simulink model "KalmanFilters"  (R2019b)
settings: Solver=FixedStepAuto  StartTime=0.0  StopTime=26.9950  FixedStep=0.005  RelTol=1e-3
InitFcn:
  | load('BusDefinitions.mat')
values from neighbouring files (symbols this model uses):
  M = [1 1 1 1 ... (first row only)    [parrot copy.m]
  q1 = 19.0085    [parrot copy.m]
  q2 = 5.761    [parrot copy.m]
  q3 = 15.4224    [parrot copy.m]
  q4 = 1.4190    (= 1.419)    [parrot copy.m]
  q5 = 6.1085    [parrot copy.m]
  r1 = .0731    (= 0.0731)    [parrot copy.m]
  r2 = 4.9726e+03    (= 4972.6)    [parrot copy.m]
  r3 = 7.7884e+03    (= 7788.4)    [parrot copy.m]
  r4 = .0160    (= 0.016)    [parrot copy.m]
  r5 = 3.0877    [parrot copy.m]
undefined symbols (not defined in the file or in its folder): codertarget, DiscIntNeverNeededParam, Discrete, Time
libraries: ctrlSharedLib x5
settings Model: ExtModeTrigDuration=80  Creator=The MathWorks, Inc.  LastModifiedBy=jockabethponce
settings DataIOCC: ReturnWorkspaceOutputs=off
settings OptimizationCC: PassReuseOutputArgsThreshold=0  MaxStackSize=64
settings DebuggingCC: ParameterTunabilityLossMsg=error  PregeneratedLibrarySubsystemCodeDiagnostic=none  ArithmeticOperatorsInVariantConditions=warning
settings HardwareCC: ProdBitPerPointer=32  ProdBitPerSizeT=32  ProdBitPerPtrDiffT=32  ProdLargestAtomicInteger=Long  ProdWordSize=32  ProdHWDeviceType=ARM Compatible->ARM 9
settings SFSimCC: SimUseLocalCustomCode=off  MATLABDynamicMemAlloc=off  CustomCodeUndefinedFunction=UseInterfaceOnly
settings RTWCC: SystemTargetFile=ert.tlc  HardwareBoard=PARROT Mambo  TLCOptions=-aInlineSetEventsForThisBaseRateFcn=TLC_FALSE -aSuppressMultiTaskScheduler=TLC_FALSE -aRateBasedStepFcn=1  TemplateMakefile=ert_default_tmf  GenerateReport=on  RTWUseLocalCustomCode=off  Toolchain=Sourcery G++ Lite GNU Toolchain for Drones  BuildConfiguration=Specify  LaunchReport=on
settings CodeAppCC: ForceParamTrailComments=on  OperatorAnnotations=on  StateflowObjectComments=on
settings ERTTargetCC: ERTCustomFileBanners=off  MatFileLogging=on  SupportContinuousTime=on  SupportNonInlinedSFcns=on  RemoveResetFunc=off  ModelStepFunctionPrototypeControlCompliant=off

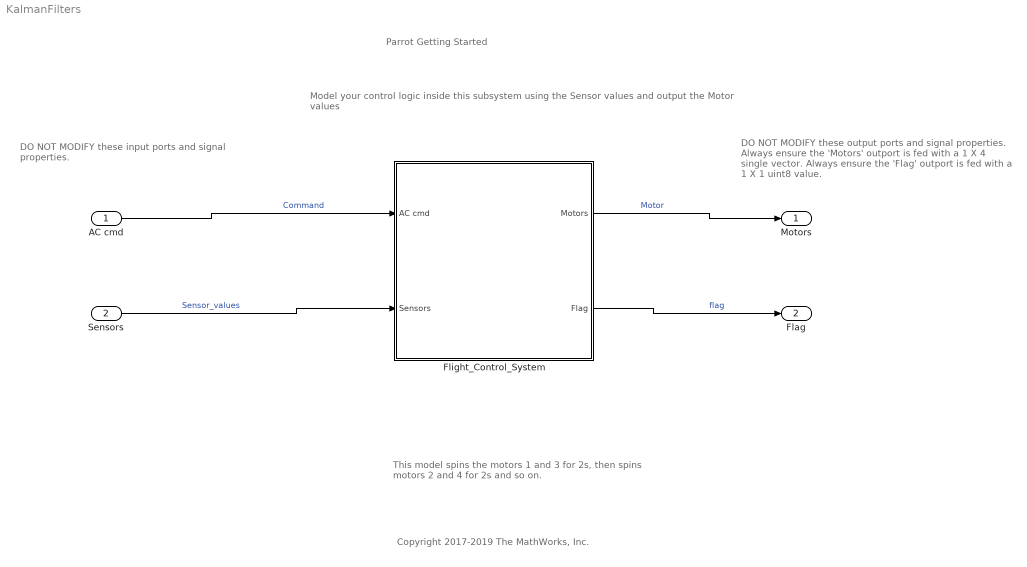
== system KalmanFilters ==
  note: Model your control logic inside this subsystem using the Sensor
      | values and output the Motor values
  note: DO NOT MODIFY these output ports and
      | signal properties.
      |
      | Always ensure the 'Motors' outport is fed
      | with a 1 X 4 single vector.
      |
      |
      |
      |
      | Always ensure the 'Flag' outport is fed
      | with a 1 X 1 uint8 value.
  note: DO NOT MODIFY these input ports and
      | signal properties.
  note: This model spins the motors 1 and 3 for 2s, then spins motors 2 and 4 for 2s and so on.
  note: Copyright 2017-2019 The MathWorks, Inc.
  note: Parrot Getting Started
  AC cmd : Inport  OutDataTypeStr=Bus: CommandBus  BusOutputAsStruct=on
  Sensors : Inport  Port=2  OutDataTypeStr=Bus: SensorsBus  BusOutputAsStruct=on
  Flight_Control_System : Subsystem  InitFcn=codertarget.parrot.internal.fcsSubsystemCallback(gcb);
  Motors : Outport  OutDataTypeStr=single  PortDimensions=[1 4]  VectorParamsAs1DForOutWhenUnconnected=off
  Flag : Outport  Port=2  OutDataTypeStr=uint8  PortDimensions=1  VectorParamsAs1DForOutWhenUnconnected=off
  wires:
  Flight_Control_System/1(Motors) -> Motors/1  "Motor"
  AC cmd/1 -> Flight_Control_System/1(AC cmd)  "Command"
  Sensors/1 -> Flight_Control_System/2(Sensors)  "Sensor_values"
  Flight_Control_System/2(Flag) -> Flag/1  "flag"

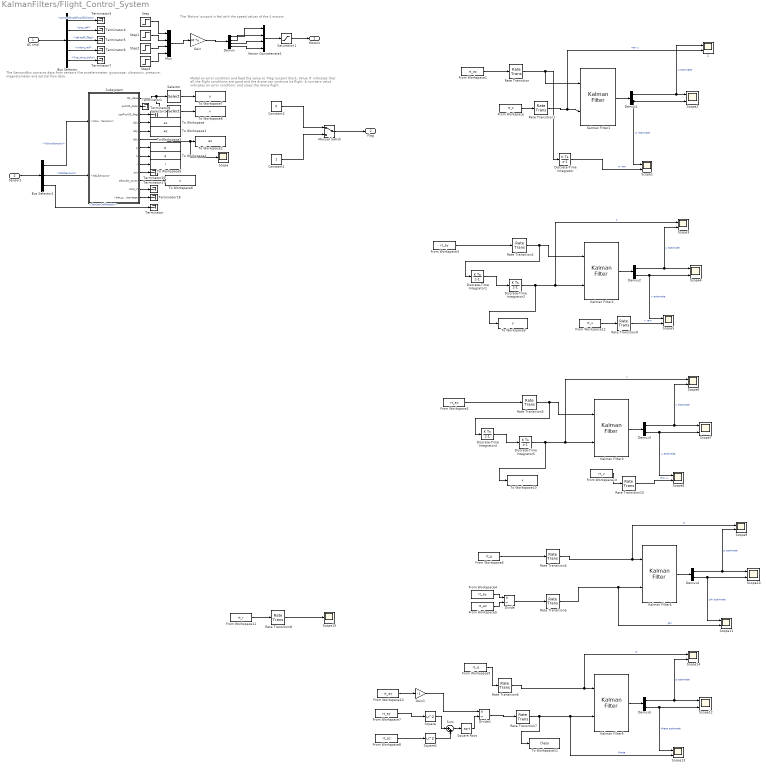
== system KalmanFilters/Flight_Control_System ==
  note: The 'Motors' outport is fed with the speed values of the 4 motors.
  note: Model an error condition and feed the value to 'Flag' outport block.
      | Value '0' indicates that all the flight conditions are good and the drone
      | can continue its flight.
      | A non-zero value indicates an error condition, and stops the drone
      | flight.
  note: The SensorsBus contains data from sensors like
      | accelerometer, gyroscope, ultrasonic, pressure,
      | magnetometer and optical flow data.
  AC cmd : Inport
  Sensors : Inport  Port=2
  Bus Selector : BusSelector  OutputSignals=controlModePosVSOrient,pos_ref,takeoff_flag,orient_ref,live_time_ticks
  Bus Selector1 : BusSelector  OutputSignals=VisionSensors,HALSensors,SensorCalibration
  Constant1 : Constant  OutDataTypeStr=uint8
  Constant2 : Constant  Value=0  OutDataTypeStr=uint8
  Demux : Demux
  Demux{1..5} (5 alike) : Demux  Outputs=2
  Discrete-Time Integrator{,1..2,4..5} (5 alike) : DiscreteIntegrator  SampleTime=.005  ICPrevOutput=DiscIntNeverNeededParam  ICPrevScaledInput=DiscIntNeverNeededParam
  Divide : Product  Inputs=*/
  Divide1 : Product  Inputs=*/
  From Workspace : FromWorkspace  VariableName=rt_z  SampleTime=.005
  From Workspace1 : FromWorkspace  VariableName=rt_az  SampleTime=.005
  From Workspace10 : FromWorkspace  VariableName=rt_ax  SampleTime=.005
  From Workspace11 : FromWorkspace  VariableName=rt_r  SampleTime=0
  From Workspace12 : FromWorkspace  VariableName=rt_v  SampleTime=0
  From Workspace13 : FromWorkspace  VariableName=rt_u  SampleTime=0
  From Workspace2 : FromWorkspace  VariableName=rt_ax  SampleTime=.005
  From Workspace3 : FromWorkspace  VariableName=rt_ay  SampleTime=.005
  From Workspace4 : FromWorkspace  VariableName=rt_ay  SampleTime=.005
  From Workspace5 : FromWorkspace  VariableName=rt_az  SampleTime=.005
  From Workspace6 : FromWorkspace  VariableName=rt_p  SampleTime=.005
  From Workspace7 : FromWorkspace  VariableName=rt_ay  SampleTime=.005
  From Workspace8 : FromWorkspace  VariableName=rt_az  SampleTime=.005
  From Workspace9 : FromWorkspace  VariableName=rt_q  SampleTime=.005
  Gain : Gain  Gain=M  Multiplication=Matrix(K*u) (u vector)
  Gain1 : Gain  Gain=-1
  Kalman Filter1 : ctrlSharedLib/Kalman Filter  TimeDomain=Discrete-Time  UseCurrentEstimator=on  ModelSource=Individual A, B, C, D matrices  ModelSourceVariable=ss(0.95,1,1,0,1)  A=[1 0.005 ; 0 1]  B="[0.005^2/2 ;  0.005]"  C=[1 0]  D=0  NumberOfStates=1  NumberOfInputs=1  NumberOfOutputs=1  InitialEstimateSource=Dialog  X0=[0;0 ]  P0=10  UseK=off  UseGH=off  NumberOfProcessNoiseInputs=1  G=1  TimeInvariantG=on  H=0  TimeInvariantH=on  Q=[0 0 ; 0 1]*q1;  TimeInvariantQ=on  R=r1  TimeInvariantR=on  N=0  TimeInvariantN=on  AddInputPort=on  AddEnablePort=off  OutputEstimatedY=off  OutputP=off  Ts=-1
      settings: SourceProductBaseCode=CT
  Kalman Filter2 : ctrlSharedLib/Kalman Filter  TimeDomain=Discrete-Time  UseCurrentEstimator=on  ModelSource=Individual A, B, C, D matrices  ModelSourceVariable=ss(0.95,1,1,0,1)  A=[1 0.005 ; 0 1]  B="[0.005^2/2 ;  0.005]"  C=[1 0]  D=0  NumberOfStates=1  NumberOfInputs=1  NumberOfOutputs=1  InitialEstimateSource=Dialog  X0=[0;0 ]  P0=10  UseK=off  UseGH=off  NumberOfProcessNoiseInputs=1  G=1  TimeInvariantG=on  H=0  TimeInvariantH=on  Q=[0 0 ; 0 1]*q2;  TimeInvariantQ=on  R=r2  TimeInvariantR=on  N=0  TimeInvariantN=on  AddInputPort=on  AddEnablePort=off  OutputEstimatedY=off  OutputP=off  Ts=-1
      settings: SourceProductBaseCode=CT
  Kalman Filter3 : ctrlSharedLib/Kalman Filter  TimeDomain=Discrete-Time  UseCurrentEstimator=on  ModelSource=Individual A, B, C, D matrices  ModelSourceVariable=ss(0.95,1,1,0,1)  A=[1 0.005 ; 0 1]  B="[0.005^2/2 ;  0.005]"  C=[1 0]  D=0  NumberOfStates=1  NumberOfInputs=1  NumberOfOutputs=1  InitialEstimateSource=Dialog  X0=[0;0 ]  P0=10  UseK=off  UseGH=off  NumberOfProcessNoiseInputs=1  G=1  TimeInvariantG=on  H=0  TimeInvariantH=on  Q=[0 0 ; 0 1]*q3;  TimeInvariantQ=on  R=r3  TimeInvariantR=on  N=0  TimeInvariantN=on  AddInputPort=on  AddEnablePort=off  OutputEstimatedY=off  OutputP=off  Ts=-1
      settings: SourceProductBaseCode=CT
  Kalman Filter4 : ctrlSharedLib/Kalman Filter  TimeDomain=Discrete-Time  UseCurrentEstimator=on  ModelSource=Individual A, B, C, D matrices  ModelSourceVariable=ss(0.95,1,1,0,1)  A=[1 0.005 ; 0 1]  B="[0.005^2/2 ;  0.005]"  C=[1 0]  D=0  NumberOfStates=1  NumberOfInputs=1  NumberOfOutputs=1  InitialEstimateSource=Dialog  X0=[0;0 ]  P0=10  UseK=off  UseGH=off  NumberOfProcessNoiseInputs=1  G=1  TimeInvariantG=on  H=0  TimeInvariantH=on  Q=[0 0 ; 0 1]*q4;  TimeInvariantQ=on  R=r4  TimeInvariantR=on  N=0  TimeInvariantN=on  AddInputPort=on  AddEnablePort=off  OutputEstimatedY=off  OutputP=off  Ts=-1
      settings: SourceProductBaseCode=CT
  Kalman Filter5 : ctrlSharedLib/Kalman Filter  TimeDomain=Discrete-Time  UseCurrentEstimator=on  ModelSource=Individual A, B, C, D matrices  ModelSourceVariable=ss(0.95,1,1,0,1)  A=[1 0.005 ; 0 1]  B="[0.005^2/2 ;  0.005]"  C=[1 0]  D=0  NumberOfStates=1  NumberOfInputs=1  NumberOfOutputs=1  InitialEstimateSource=Dialog  X0=[0;0 ]  P0=10  UseK=off  UseGH=off  NumberOfProcessNoiseInputs=1  G=1  TimeInvariantG=on  H=0  TimeInvariantH=on  Q=[0 0 ; 0 1]*q5;  TimeInvariantQ=on  R=r5  TimeInvariantR=on  N=0  TimeInvariantN=on  AddInputPort=on  AddEnablePort=off  OutputEstimatedY=off  OutputP=off  Ts=-1
      settings: SourceProductBaseCode=CT
  Manual Switch : ManualSwitch
  Mux : Mux
  Rate Transition{,1..10} (11 alike) : RateTransition  OutPortSampleTime=.005
  Saturation1 : Saturate  UpperLimit=500  LowerLimit=-500  OutDataTypeStr=single
  Scope : Scope
  Scope{1..14} (14 alike) : Scope  NumInputPorts=2
  Scope15 : Scope
  Selector : Selector  InputPortWidth=3  IndexOptions=Index vector (dialog)  Indices=[1]  OutputSizes=1
  Selector1 : Selector  InputPortWidth=3  IndexOptions=Index vector (dialog)  Indices=[2]  OutputSizes=1
  Square : Math  Operator=square  SignedPower=off  SaturateOnIntegerOverflow=on
  Square Root : Sqrt  SaturateOnIntegerOverflow=on
  Square1 : Math  Operator=square  SignedPower=off  SaturateOnIntegerOverflow=on
  Step{,1..3} (4 alike) : Step  After=0  SampleTime=.005
  Subsystem : Subsystem
  Sum : Sum  Inputs=|++
  Terminator{,1,3..8,15,17..18} (11 alike) : Terminator
  To Workspace : ToWorkspace  VariableName=ax  SaveFormat=Structure With Time  SampleTime=-1
  To Workspace1 : ToWorkspace  VariableName=ay  SaveFormat=Structure With Time  SampleTime=-1
  To Workspace10 : ToWorkspace  VariableName=x  SaveFormat=Timeseries  SampleTime=-1
  To Workspace11 : ToWorkspace  VariableName=theta  SaveFormat=Timeseries  SampleTime=.005
  To Workspace2 : ToWorkspace  VariableName=az  SaveFormat=Structure With Time  SampleTime=-1
  To Workspace3 : ToWorkspace  VariableName=p  SaveFormat=Structure With Time  SampleTime=-1
  To Workspace4 : ToWorkspace  VariableName=q  SaveFormat=Structure With Time  SampleTime=-1
  To Workspace5 : ToWorkspace  VariableName=r  SaveFormat=Structure With Time  SampleTime=-1
  To Workspace6 : ToWorkspace  VariableName=z  SaveFormat=Structure With Time  SampleTime=-1
  To Workspace7 : ToWorkspace  VariableName=u  SaveFormat=Structure With Time  SampleTime=-1
  To Workspace8 : ToWorkspace  VariableName=v  SaveFormat=Structure With Time  SampleTime=-1
  To Workspace9 : ToWorkspace  VariableName=y  SaveFormat=Timeseries  SampleTime=-1
  Vector Concatenate1 : Concatenate  NumInputs=4
  z : Scope  NumInputPorts=2
  Motors : Outport  VectorParamsAs1DForOutWhenUnconnected=off
  Flag : Outport  Port=2  VectorParamsAs1DForOutWhenUnconnected=off
  wires:
  AC cmd/1 -> Bus Selector/1
  Bus Selector/1 -> Terminator3/1  "<controlModePosVSOrient>"
  Bus Selector/2 -> Terminator4/1  "<pos_ref>"
  Bus Selector/3 -> Terminator5/1  "<takeoff_flag>"
  Bus Selector/4 -> Terminator6/1  "<orient_ref>"
  Bus Selector/5 -> Terminator7/1  "<live_time_ticks>"
  Manual Switch/1 -> Flag/1
  Constant2/1 -> Manual Switch/1
  Constant1/1 -> Manual Switch/2
  Saturation1/1 -> Motors/1
  Vector Concatenate1/1 -> Saturation1/1
  Subsystem/8(q) -> To Workspace4/1
  Subsystem/13(vbat_percentage) -> Terminator18/1
  Bus Selector1/3 -> Terminator/1  "<SensorCalibration>"
  Subsystem/10(prs) -> Terminator15/1
  Bus Selector1/2 -> Subsystem/2(<HALSensors>)  "<HALSensors>"
  Bus Selector1/1 -> Subsystem/1(<VisionSensors>)  "<VisionSensors>"
  Subsystem/9(r) -> To Workspace5/1
  Subsystem/1(OF_data) -> Selector1/1, Selector/1
  Subsystem/3(usePosVIS_flag) -> Terminator8/1
  Subsystem/6(ddz) -> Scope/1, To Workspace2/1
  Subsystem/5(ddy) -> To Workspace1/1
  Subsystem/11(altitude_sonar) -> To Workspace6/1
  Subsystem/12(vbat_V) -> Terminator17/1
  Subsystem/4(ddx) -> To Workspace/1
  Subsystem/7(p) -> To Workspace3/1
  Sensors/1 -> Bus Selector1/1
  Step2/1 -> Mux/3
  Step/1 -> Mux/1
  Step1/1 -> Mux/2
  Step3/1 -> Mux/4
  Mux/1 -> Gain/1
  Gain/1 -> Demux/1
  Demux/1 -> Vector Concatenate1/1
  Demux/2 -> Vector Concatenate1/2
  Demux/3 -> Vector Concatenate1/3
  Demux/4 -> Vector Concatenate1/4
  Selector/1 -> To Workspace7/1
  Selector1/1 -> To Workspace8/1
  Subsystem/2(posVIS_data) -> Terminator1/1
  Kalman Filter1/1 -> Demux1/1
  Demux1/1 -> z/1, Scope2/1  "z estimate"
  From Workspace1/1 -> Rate Transition/1
  From Workspace/1 -> Rate Transition1/1
  Rate Transition1/1 -> z/2, Kalman Filter1/2  "raw z"
  Demux1/2 -> Scope1/1, Scope2/2  "w estimate"
  Rate Transition/1 -> Discrete-Time Integrator/1, Kalman Filter1/1
  Discrete-Time Integrator/1 -> Scope1/2  "w raw"
  Demux2/2 -> Scope5/1, Scope4/2  "v estimate"
  Kalman Filter2/1 -> Demux2/1
  Demux2/1 -> Scope3/2, Scope4/1  "y estimate"
  Rate Transition2/1 -> Discrete-Time Integrator1/1, Kalman Filter2/1
  Discrete-Time Integrator1/1 -> Discrete-Time Integrator2/1
  Discrete-Time Integrator2/1 -> To Workspace9/1, Scope3/1, Kalman Filter2/2  "y"
  From Workspace3/1 -> Rate Transition2/1
  Discrete-Time Integrator5/1 -> To Workspace10/1, Scope6/1, Kalman Filter3/2  "x"
  Discrete-Time Integrator4/1 -> Discrete-Time Integrator5/1
  Demux3/1 -> Scope6/2, Scope7/1  "x estimate"
  From Workspace2/1 -> Rate Transition3/1
  Demux3/2 -> Scope8/1, Scope7/2  "u estimate"
  Kalman Filter3/1 -> Demux3/1
  Rate Transition3/1 -> Discrete-Time Integrator4/1, Kalman Filter3/1
  Demux4/1 -> Scope9/2, Scope10/1  "p estimate"
  Demux4/2 -> Scope11/1, Scope10/2  "phi estimate"
  Kalman Filter4/1 -> Demux4/1
  From Workspace4/1 -> Divide/1
  From Workspace5/1 -> Divide/2
  Divide/1 -> Rate Transition5/1
  From Workspace6/1 -> Rate Transition4/1
  Rate Transition4/1 -> Scope9/1, Kalman Filter4/1  "p"
  Rate Transition5/1 -> Scope11/2, Kalman Filter4/2  "phi"
  Rate Transition7/1 -> To Workspace11/1, Scope13/2, Kalman Filter5/2  "theta"
  Kalman Filter5/1 -> Demux5/1
  Rate Transition6/1 -> Scope14/1, Kalman Filter5/1  "q"
  Demux5/1 -> Scope14/2, Scope12/1  "q estimate"
  Demux5/2 -> Scope13/1, Scope12/2  "theta estimate"
  From Workspace9/1 -> Rate Transition6/1
  From Workspace7/1 -> Square/1
  From Workspace8/1 -> Square1/1
  Square/1 -> Sum/1
  Square1/1 -> Sum/2
  Sum/1 -> Square Root/1
  From Workspace10/1 -> Gain1/1
  Gain1/1 -> Divide1/1
  Square Root/1 -> Divide1/2
  Divide1/1 -> Rate Transition7/1
  From Workspace11/1 -> Rate Transition8/1
  Rate Transition8/1 -> Scope15/1
  Rate Transition9/1 -> Scope5/2  "v raw"
  From Workspace13/1 -> Rate Transition10/1
  Rate Transition10/1 -> Scope8/2  "raw u"
  From Workspace12/1 -> Rate Transition9/1

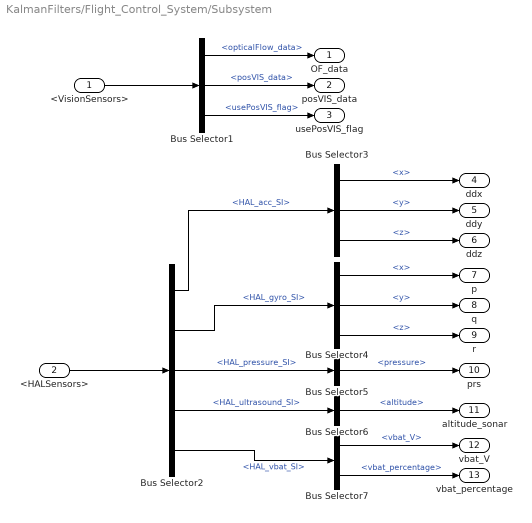
== system KalmanFilters/Flight_Control_System/Subsystem ==
  <VisionSensors> : Inport
  <HALSensors> : Inport  Port=2
  Bus Selector1 : BusSelector  OutputSignals=opticalFlow_data,posVIS_data,usePosVIS_flag
  Bus Selector2 : BusSelector  OutputSignals=HAL_acc_SI,HAL_gyro_SI,HAL_pressure_SI,HAL_ultrasound_SI,HAL_vbat_SI
  Bus Selector3 : BusSelector  OutputSignals=x,y,z
  Bus Selector4 : BusSelector  OutputSignals=x,y,z
  Bus Selector5 : BusSelector  OutputSignals=pressure
  Bus Selector6 : BusSelector  OutputSignals=altitude
  Bus Selector7 : BusSelector  OutputSignals=vbat_V,vbat_percentage
  OF_data : Outport  VectorParamsAs1DForOutWhenUnconnected=off
  posVIS_data : Outport  Port=2  VectorParamsAs1DForOutWhenUnconnected=off
  usePosVIS_flag : Outport  Port=3  VectorParamsAs1DForOutWhenUnconnected=off
  ddx : Outport  Port=4  VectorParamsAs1DForOutWhenUnconnected=off
  ddy : Outport  Port=5  VectorParamsAs1DForOutWhenUnconnected=off
  ddz : Outport  Port=6  VectorParamsAs1DForOutWhenUnconnected=off
  p : Outport  Port=7  VectorParamsAs1DForOutWhenUnconnected=off
  q : Outport  Port=8  VectorParamsAs1DForOutWhenUnconnected=off
  r : Outport  Port=9  VectorParamsAs1DForOutWhenUnconnected=off
  prs : Outport  Port=10  VectorParamsAs1DForOutWhenUnconnected=off
  altitude_sonar : Outport  Port=11  VectorParamsAs1DForOutWhenUnconnected=off
  vbat_V : Outport  Port=12  VectorParamsAs1DForOutWhenUnconnected=off
  vbat_percentage : Outport  Port=13  VectorParamsAs1DForOutWhenUnconnected=off
  wires:
  <VisionSensors>/1 -> Bus Selector1/1
  <HALSensors>/1 -> Bus Selector2/1
  Bus Selector1/1 -> OF_data/1  "<opticalFlow_data>"
  Bus Selector1/2 -> posVIS_data/1  "<posVIS_data>"
  Bus Selector1/3 -> usePosVIS_flag/1  "<usePosVIS_flag>"
  Bus Selector2/1 -> Bus Selector3/1  "<HAL_acc_SI>"
  Bus Selector2/2 -> Bus Selector4/1  "<HAL_gyro_SI>"
  Bus Selector2/3 -> Bus Selector5/1  "<HAL_pressure_SI>"
  Bus Selector2/4 -> Bus Selector6/1  "<HAL_ultrasound_SI>"
  Bus Selector2/5 -> Bus Selector7/1  "<HAL_vbat_SI>"
  Bus Selector3/1 -> ddx/1  "<x>"
  Bus Selector3/2 -> ddy/1  "<y>"
  Bus Selector3/3 -> ddz/1  "<z>"
  Bus Selector4/2 -> q/1  "<y>"
  Bus Selector4/1 -> p/1  "<x>"
  Bus Selector4/3 -> r/1  "<z>"
  Bus Selector5/1 -> prs/1  "<pressure>"
  Bus Selector6/1 -> altitude_sonar/1  "<altitude>"
  Bus Selector7/1 -> vbat_V/1  "<vbat_V>"
  Bus Selector7/2 -> vbat_percentage/1  "<vbat_percentage>"
